simulink model "EchoEffect"  (R2020a)
settings: Solver=VariableStepAuto  StartTime=0.0  StopTime=50  RelTol=1e-3
libraries: dspsnks4 x1, dspvision x1, simulink x1
settings Model: Creator=Administrator  LastModifiedBy=Administrator

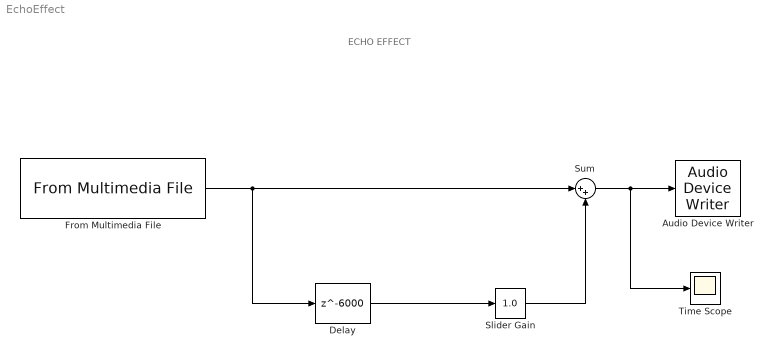
== system EchoEffect ==
  note: ECHO EFFECT
  Audio Device Writer : dspsnks4/Audio Device Writer  Driver=DirectSound  Device=Default  InheritSampleRate=on  SampleRate=44100  BitDepth=16-bit integer  BufferSize=4096  NumBuffers=10  DefaultOutputChannelMapping=on  OutputChannelMapping=1:2  OutputNumUnderrunSamples=off  DriverIdx=1  DeviceWarnFlag=''
  Delay : Delay  DelayLength=6000  InitialCondition=0  InputProcessing=Columns as channels (frame based)  UseCircularBuffer=on
  From Multimedia File : dspvision/From Multimedia File  inputFilename=C:\Users\Administrator\Downloads\countdown-ten-seconds-76982.mp3  readRange=[1 Inf]  loop=on  numPlays=inf  outputStreams=Audio only  videoDataType=single  audioDataType=double  inheritSampleTime=on  userDefinedSampleTime=1/30  noAudioOutput=off  isIntensityVideo=off  fourcc=RGB  colorVideoFormat=Separate color signals  outputEOF=off  dataOrg=Column-major  audioFrameSize=1024  computeAudioFrameSize=off  outSamplingMode=Sample based
  Slider Gain : simulink/Math Operations/Slider Gain  gain=1.0  low=0  high=1
  Sum : Sum  Inputs=|++
  Time Scope : Scope
  wires:
  Delay/1 -> Slider Gain/1
  From Multimedia File/1 -> Sum/1, Delay/1
  Sum/1 -> Time Scope/1, Audio Device Writer/1
  Slider Gain/1 -> Sum/2
